simulink model "ARINC429_BNR"  (R2020b)
settings: Solver=VariableStepAuto  StartTime=0.0  StopTime=10.0  RelTol=1e-3
libraries: Bibavion x1
(part 3 of 3)

== system ARINC429_BNR/Decoder/Decode/C2 Decoder/De-serialize/Subsystem2 ==
  In1 : Inport
  Data Type Conversion5 : DataTypeConversion  OutDataTypeStr=uint32
  Data Type Conversion9 : DataTypeConversion  OutDataTypeStr=uint32
  Divide12 : Product  Inputs=*/  OutDataTypeStr=double
  Divide13 : Product  Inputs=*/  OutDataTypeStr=uint32
  Float Const : Constant  Value=2  OutDataTypeStr=single
  Float Const6 : Constant  Value=0.5  OutDataTypeStr=single
  Subtract5 : Sum  Inputs=+-
  Out1 : Outport
  Out2 : Outport  Port=2
  wires:
  Float Const/1 -> [F_2]
  Divide12/1 -> Subtract5/1, Data Type Conversion5/1
  Divide13/1 -> Data Type Conversion9/1
  Float Const6/1 -> Divide13/2
  Data Type Conversion5/1 -> Out2/1, Subtract5/2
  [F_2] -> Divide12/2
  Subtract5/1 -> Divide13/1
  Data Type Conversion9/1 -> Out1/1
  In1/1 -> Divide12/1

== system ARINC429_BNR/Decoder/Decode/C2 Decoder/De-serialize/Subsystem3 ==
  In1 : Inport
  Data Type Conversion5 : DataTypeConversion  OutDataTypeStr=uint32
  Data Type Conversion9 : DataTypeConversion  OutDataTypeStr=uint32
  Divide12 : Product  Inputs=*/  OutDataTypeStr=double
  Divide13 : Product  Inputs=*/
  Float Const : Constant  Value=2  OutDataTypeStr=single
  Float Const6 : Constant  Value=0.5  OutDataTypeStr=single
  Subtract5 : Sum  Inputs=+-
  Out1 : Outport
  Out2 : Outport  Port=2
  wires:
  Float Const/1 -> [F_2]
  Divide12/1 -> Subtract5/1, Data Type Conversion5/1
  Divide13/1 -> Data Type Conversion9/1
  Float Const6/1 -> Divide13/2
  Data Type Conversion5/1 -> Out2/1, Subtract5/2
  In1/1 -> Divide12/1
  [F_2] -> Divide12/2
  Subtract5/1 -> Divide13/1
  Data Type Conversion9/1 -> Out1/1

== system ARINC429_BNR/Decoder/Decode/C2 Decoder/De-serialize/Subsystem4 ==
  In1 : Inport
  Data Type Conversion5 : DataTypeConversion  OutDataTypeStr=uint32
  Data Type Conversion9 : DataTypeConversion  OutDataTypeStr=uint32
  Divide12 : Product  Inputs=*/  OutDataTypeStr=double
  Divide13 : Product  Inputs=*/  OutDataTypeStr=uint32
  Float Const : Constant  Value=2  OutDataTypeStr=single
  Float Const6 : Constant  Value=0.5  OutDataTypeStr=single
  Subtract5 : Sum  Inputs=+-
  Out1 : Outport
  Out2 : Outport  Port=2
  wires:
  Float Const/1 -> [F_2]
  Divide12/1 -> Subtract5/1, Data Type Conversion5/1
  Divide13/1 -> Data Type Conversion9/1
  Float Const6/1 -> Divide13/2
  Data Type Conversion5/1 -> Out2/1, Subtract5/2
  [F_2] -> Divide12/2
  Subtract5/1 -> Divide13/1
  Data Type Conversion9/1 -> Out1/1
  In1/1 -> Divide12/1

== system ARINC429_BNR/Decoder/Decode/C2 Decoder/De-serialize/Subsystem7 ==
  In1 : Inport
  Data Type Conversion5 : DataTypeConversion  OutDataTypeStr=uint32
  Data Type Conversion9 : DataTypeConversion  OutDataTypeStr=uint32
  Divide12 : Product  Inputs=*/  OutDataTypeStr=double
  Divide13 : Product  Inputs=*/  OutDataTypeStr=uint32
  Float Const : Constant  Value=2  OutDataTypeStr=single
  Float Const6 : Constant  Value=0.5  OutDataTypeStr=single
  Subtract5 : Sum  Inputs=+-
  Out1 : Outport
  Out2 : Outport  Port=2
  wires:
  Float Const/1 -> [F_2]
  Divide12/1 -> Subtract5/1, Data Type Conversion5/1
  Divide13/1 -> Data Type Conversion9/1
  Float Const6/1 -> Divide13/2
  Data Type Conversion5/1 -> Out2/1, Subtract5/2
  [F_2] -> Divide12/2
  Subtract5/1 -> Divide13/1
  Data Type Conversion9/1 -> Out1/1
  In1/1 -> Divide12/1

== system ARINC429_BNR/Decoder/Decode/C2 Decoder/De-serialize/Subsystem8 ==
  In1 : Inport
  Data Type Conversion5 : DataTypeConversion  OutDataTypeStr=uint32
  Data Type Conversion9 : DataTypeConversion  OutDataTypeStr=uint32
  Divide12 : Product  Inputs=*/  OutDataTypeStr=double
  Divide13 : Product  Inputs=*/  OutDataTypeStr=uint32
  Float Const : Constant  Value=2  OutDataTypeStr=single
  Float Const6 : Constant  Value=0.5  OutDataTypeStr=single
  Subtract5 : Sum  Inputs=+-
  Out1 : Outport
  Out2 : Outport  Port=2
  wires:
  Float Const/1 -> [F_2]
  Divide12/1 -> Subtract5/1, Data Type Conversion5/1
  Divide13/1 -> Data Type Conversion9/1
  Float Const6/1 -> Divide13/2
  Data Type Conversion5/1 -> Out2/1, Subtract5/2
  [F_2] -> Divide12/2
  Subtract5/1 -> Divide13/1
  Data Type Conversion9/1 -> Out1/1
  In1/1 -> Divide12/1

== system ARINC429_BNR/Decoder/Decode/C2 Decoder/De-serialize/Subsystem9 ==
  In1 : Inport
  Data Type Conversion5 : DataTypeConversion  OutDataTypeStr=uint32
  Data Type Conversion9 : DataTypeConversion  OutDataTypeStr=uint32
  Divide12 : Product  Inputs=*/  OutDataTypeStr=double
  Divide13 : Product  Inputs=*/  OutDataTypeStr=uint32
  Float Const : Constant  Value=2  OutDataTypeStr=single
  Float Const6 : Constant  Value=0.5  OutDataTypeStr=single
  Subtract5 : Sum  Inputs=+-
  Out1 : Outport
  Out2 : Outport  Port=2
  wires:
  Float Const/1 -> [F_2]
  Divide12/1 -> Subtract5/1, Data Type Conversion5/1
  Divide13/1 -> Data Type Conversion9/1
  Float Const6/1 -> Divide13/2
  Data Type Conversion5/1 -> Out2/1, Subtract5/2
  [F_2] -> Divide12/2
  Subtract5/1 -> Divide13/1
  Data Type Conversion9/1 -> Out1/1
  In1/1 -> Divide12/1
